simulink model "SingleTrackCANoe"  (R2021b)
settings: Solver=ode1  StartTime=0  StopTime=2  FixedStep=1.0000000000000000e-003  RelTol=1e-3
InitFcn:
  | sampleTime = str2double(get_param(bdroot, 'FixedStep'));
undefined symbols (not defined in the file or in its folder): AccPedalPos, BrakePedalPos, BrakeSwitch, DiscIntNeverNeededParam, DYNA4, EngSpd, IgnitionSwitch, InitialGear, InitialSpeed, IntendedEngTrq, LeftIndicator, MainBrakePress, MaxGear, MDL, MinGear, RefAcc, RefLane, RefLatPos, RefPath, RefPathCurv, RefSpd, RefSpdPreview, RefSpdRetrospect, RightIndicator, SteeringWheelAng, SteeringWheelTrq, UserDefinedRefValue, vm_const
libraries: UtilitiesLibrary x62, simulink x18, WheelSystemModules x14, LongitudinalControllerModules x13, LateralControllerModules x7, AnimationBusselectorModules x5, EnvironmentModules x5, BasicEngineControlModules x5, MiscellaneousControlModules x5, Animation3Modules x4, AuxiliariesModules x4, ReducedTireModules x4
(part 10 of 34)

== system SingleTrackCANoe/SimulationModel/VehicleControl/VehicleControlOutput ==
  InitialConditions___UNIQUE_1 : Inport  Description=|
      | <name>InitialConditions</name>
      | <comment></comment>
  LongitudinalControl___UNIQUE_1 : Inport  Description=|  Port=2
      | <name>LongitudinalControl</name>
      | <comment></comment>
  LateralControl___UNIQUE_1 : Inport  Description=|  Port=3
      | <name>LateralControl</name>
      | <comment></comment>
  BrakeHydraulicsControl___UNIQUE_1 : Inport  Description=|  Port=4
      | <name>BrakeHydraulicsControl</name>
      | <comment></comment>
  EngineControl___UNIQUE_1 : Inport  Description=|  Port=5
      | <name>EngineControl</name>
      | <comment></comment>
  SuspensionTestRigControl___UNIQUE_1 : Inport  Description=|  Port=6
      | <name>SuspensionTestRigControl</name>
      | <comment></comment>
  TemperatureControl___UNIQUE_1 : Inport  Description=|  Port=7
      | <name>TemperatureControl</name>
      | <comment></comment>
  UserDefinedControl___UNIQUE_1 : Inport  Description=|  Port=8
      | <name>UserDefinedControl</name>
      | <comment></comment>
  __TDO__VehicleControl : BusCreator  Inputs=8
  VehicleControl___UNIQUE_1 : Outport  Description=|  VectorParamsAs1DForOutWhenUnconnected=off
      | <name>InitialConditions</name>
      | <comment></comment>
  wires:
  InitialConditions___UNIQUE_1/1 -> __TDO__VehicleControl/1  "InitialConditions"
  LongitudinalControl___UNIQUE_1/1 -> __TDO__VehicleControl/2  "LongitudinalControl"
  LateralControl___UNIQUE_1/1 -> __TDO__VehicleControl/3  "LateralControl"
  BrakeHydraulicsControl___UNIQUE_1/1 -> __TDO__VehicleControl/4  "BrakeHydraulicsControl"
  EngineControl___UNIQUE_1/1 -> __TDO__VehicleControl/5  "EngineControl"
  SuspensionTestRigControl___UNIQUE_1/1 -> __TDO__VehicleControl/6  "SuspensionTestRigControl"
  TemperatureControl___UNIQUE_1/1 -> __TDO__VehicleControl/7  "TemperatureControl"
  UserDefinedControl___UNIQUE_1/1 -> __TDO__VehicleControl/8  "UserDefinedControl"
  __TDO__VehicleControl/1 -> VehicleControl___UNIQUE_1/1  "VehicleControl"

== system SingleTrackCANoe/SimulationModel/ControlUnits/ADAS/ADASOutput ==
  __SRC__ADAS.LongitudinalControlIntervention[0;1] : Constant  Value=0.0  OutDataTypeStr=Inherit: Inherit via back propagation
  __SRC__ADAS.PrioritizedADASControl.LimitsActive[0;1] : Constant  Value=0.0  OutDataTypeStr=Inherit: Inherit via back propagation
  __SRC__ADAS.PrioritizedADASControl.LowerLimitBrakePress[Pa] : Constant  Value=0.0  OutDataTypeStr=Inherit: Inherit via back propagation
  __SRC__ADAS.PrioritizedADASControl.LowerLimitTrq[Nm] : Constant  Value=-vm_const('PAR_NOT_GIVEN')  OutDataTypeStr=Inherit: Inherit via back propagation
  __SRC__ADAS.PrioritizedADASControl.UpperLimitTrq[Nm] : Constant  Value=vm_const('PAR_NOT_GIVEN')  OutDataTypeStr=Inherit: Inherit via back propagation
  __TDO__ADAS : BusCreator  Inputs=2
  __TDO__ADAS.PrioritizedADASControl : BusCreator  Inputs=4
  ADAS___UNIQUE_1 : Outport  Description=|  PortDimensions=[5]  VectorParamsAs1DForOutWhenUnconnected=off
      | <name>PrioritizedADASControl.LimitsActive[0;1]</name>
      | <comment></comment>
  wires:
  __SRC__ADAS.PrioritizedADASControl.LimitsActive[0;1]/1 -> __TDO__ADAS.PrioritizedADASControl/1  "LimitsActive[0;1]"
  __TDO__ADAS.PrioritizedADASControl/1 -> __TDO__ADAS/1  "PrioritizedADASControl"
  __SRC__ADAS.PrioritizedADASControl.UpperLimitTrq[Nm]/1 -> __TDO__ADAS.PrioritizedADASControl/2  "UpperLimitTrq[Nm]"
  __SRC__ADAS.PrioritizedADASControl.LowerLimitTrq[Nm]/1 -> __TDO__ADAS.PrioritizedADASControl/3  "LowerLimitTrq[Nm]"
  __SRC__ADAS.PrioritizedADASControl.LowerLimitBrakePress[Pa]/1 -> __TDO__ADAS.PrioritizedADASControl/4  "LowerLimitBrakePress[Pa]"
  __SRC__ADAS.LongitudinalControlIntervention[0;1]/1 -> __TDO__ADAS/2  "LongitudinalControlIntervention[0;1]"
  __TDO__ADAS/1 -> ADAS___UNIQUE_1/1  "ADAS"

== system SingleTrackCANoe/SimulationModel/ControlUnits/ADAS/DynaComponentInfo ==

== system SingleTrackCANoe/SimulationModel/ControlUnits/LCU/DynaComponentInfo ==

== system SingleTrackCANoe/SimulationModel/ControlUnits/LCU/LCUOutput ==
  VehicleLights___UNIQUE_1 : Inport  Description=|
      | <name>VehicleLights</name>
      | <comment></comment>
  __TDO__LCU : BusCreator  Inputs=1
  LCU___UNIQUE_1 : Outport  Description=|  VectorParamsAs1DForOutWhenUnconnected=off
      | <name>VehicleLights</name>
      | <comment></comment>
  wires:
  VehicleLights___UNIQUE_1/1 -> __TDO__LCU/1  "VehicleLights"
  __TDO__LCU/1 -> LCU___UNIQUE_1/1  "LCU"

== system SingleTrackCANoe/SimulationModel/ControlUnits/StateSensors/DynaComponentInfo ==

== system SingleTrackCANoe/SimulationModel/ControlUnits/StateSensors/StateSensorsOutput ==
  IMU___UNIQUE_1 : Inport  Description=|
      | <name>IMU</name>
      | <comment></comment>
  __TDO__StateSensors : BusCreator  Inputs=1
  StateSensors___UNIQUE_1 : Outport  Description=|  VectorParamsAs1DForOutWhenUnconnected=off
      | <name>IMU</name>
      | <comment></comment>
  wires:
  IMU___UNIQUE_1/1 -> __TDO__StateSensors/1  "IMU"
  __TDO__StateSensors/1 -> StateSensors___UNIQUE_1/1  "StateSensors"

== system SingleTrackCANoe/SimulationModel/ControlUnits/VCU/DynaComponentInfo ==

== system SingleTrackCANoe/SimulationModel/ControlUnits/VCU/InputFromADAS ==
  fromADAS : Inport  Description=|
      | <name>DriverBrakePedalMode[0;1;2]</name>
      | <comment></comment>
  TDBusSelector : BusSelector  OutputSignals=PrioritizedADASControl
  __TDO__PrioritizedADASControl : BusCreator  Inputs=1
  PrioritizedADASControl___UNIQUE_1 : Outport  Description=|
      | <name>PrioritizedADASControl</name>
      | <comment></comment>
  wires:
  fromADAS/1 -> TDBusSelector/1  "ControlSignals"
  TDBusSelector/1 -> __TDO__PrioritizedADASControl/1  "<PrioritizedADASControl>"
  __TDO__PrioritizedADASControl/1 -> PrioritizedADASControl___UNIQUE_1/1  "PrioritizedADASControl"

== system SingleTrackCANoe/SimulationModel/ControlUnits/VCU/InputFromCTRL ==
  fromCTRL : Inport
  TDBusSelector : BusSelector  OutputSignals=CTRL.LongitudinalControl.AccPedalPos[0_1],CTRL.LongitudinalControl.BrakePedalPos[0_1],CTRL.LongitudinalControl.DriverInfo.MeanEngMaxTrq[Nm],CTRL.LongitudinalControl.DriverInfo.MeanEngDragTrq[Nm],CTRL.LongitudinalControl.DriverInfo.ThirtyPercentAccPedalEngTrq[Nm]
  __TDD__AccPedalPos[0_1] : Demux  Outputs=[1]
  __TDD__BrakePedalPos[0_1] : Demux  Outputs=1
  __TDD__MeanEngDragTrq[Nm] : Demux  Outputs=[1]
  __TDD__MeanEngMaxTrq[Nm] : Demux  Outputs=[1]
  __TDD__ThirtyPercentAccPedalEngTrq[Nm] : Demux  Outputs=[1]
  AccPedalPos[0_1] : Outport  Description=|  PortDimensions=[1]  VectorParamsAs1DForOutWhenUnconnected=off
      | <name>CTRL.LongitudinalControl.AccPedalPos[0_1]</name>
      | <comment>Accelerator pedal position</comment>
  BrakePedalPos[0_1]___UNIQUE_1 : Outport  Description=|  Port=2  VectorParamsAs1DForOutWhenUnconnected=off
      | <name>CTRL.LongitudinalControl.BrakePedalPos[0_1]</name>
      | <comment></comment>
  MeanEngMaxTrq[Nm]___UNIQUE_1 : Outport  Description=|  Port=3  PortDimensions=[1]  VectorParamsAs1DForOutWhenUnconnected=off
      | <name>CTRL.LongitudinalControl.DriverInfo.MeanEngMaxTrq[Nm]</name>
      | <comment></comment>
  MeanEngDragTrq[Nm]___UNIQUE_1 : Outport  Description=|  Port=4  PortDimensions=[1]  VectorParamsAs1DForOutWhenUnconnected=off
      | <name>CTRL.LongitudinalControl.DriverInfo.MeanEngDragTrq[Nm]</name>
      | <comment></comment>
  ThirtyPercentAccPedalEngTrq[Nm]___UNIQUE_1 : Outport  Description=|  Port=5  PortDimensions=[1]
      | <name>CTRL.LongitudinalControl.DriverInfo.ThirtyPercentAccPedalEngTrq[Nm]</name>
      | <comment></comment>
  wires:
  __TDD__ThirtyPercentAccPedalEngTrq[Nm]/1 -> ThirtyPercentAccPedalEngTrq[Nm]___UNIQUE_1/1  "ThirtyPercentAccPedalEngTrq[Nm]"
  __TDD__MeanEngDragTrq[Nm]/1 -> MeanEngDragTrq[Nm]___UNIQUE_1/1  "MeanEngDragTrq[Nm]"
  __TDD__MeanEngMaxTrq[Nm]/1 -> MeanEngMaxTrq[Nm]___UNIQUE_1/1  "MeanEngMaxTrq[Nm]"
  __TDD__BrakePedalPos[0_1]/1 -> BrakePedalPos[0_1]___UNIQUE_1/1  "BrakePedalPos[0_1]"
  __TDD__AccPedalPos[0_1]/1 -> AccPedalPos[0_1]/1  "AccPedalPos[0_1]"
  TDBusSelector/5 -> __TDD__ThirtyPercentAccPedalEngTrq[Nm]/1  "<ThirtyPercentAccPedalEngTrq[Nm]>"
  TDBusSelector/4 -> __TDD__MeanEngDragTrq[Nm]/1  "<MeanEngDragTrq[Nm]>"
  TDBusSelector/3 -> __TDD__MeanEngMaxTrq[Nm]/1  "<MeanEngMaxTrq[Nm]>"
  TDBusSelector/2 -> __TDD__BrakePedalPos[0_1]/1  "<BrakePedalPos[0_1]>"
  TDBusSelector/1 -> __TDD__AccPedalPos[0_1]/1  "<AccPedalPos[0_1]>"
  fromCTRL/1 -> TDBusSelector/1

== system SingleTrackCANoe/SimulationModel/ControlUnits/VCU/InputFromVehicle ==
  fromVehicle : Inport
  TDBusSelector : BusSelector  OutputSignals=BrakeSystem.BrakeSystemPhysics.MaxMainBrakePress[Pa]
  __TDD__MaxMainBrakePress[Pa] : Demux  Outputs=[1]
  MaxMainBrakePress[Pa]___UNIQUE_1 : Outport  Description=|  PortDimensions=[1]  VectorParamsAs1DForOutWhenUnconnected=off
      | <name>BrakeSystem.BrakeSystemPhysics.MaxMainBrakePress[Pa]</name>
      | <comment>Maximum main brake pressure</comment>
  wires:
  fromVehicle/1 -> TDBusSelector/1
  TDBusSelector/1 -> __TDD__MaxMainBrakePress[Pa]/1  "<MaxMainBrakePress[Pa]>"
  __TDD__MaxMainBrakePress[Pa]/1 -> MaxMainBrakePress[Pa]___UNIQUE_1/1  "MaxMainBrakePress[Pa]"

== system SingleTrackCANoe/SimulationModel/ControlUnits/VCU/VCUOutput ==
  TransmissionLoad[0_1]___UNIQUE_1 : Inport  Description=|  PortDimensions=[1]
      | <name>TransmissionLoad[0_1]</name>
      | <comment></comment>
  IntendedEngTrq[Nm]___UNIQUE_1 : Inport  Description=|  Port=2  PortDimensions=[1]
      | <name>IntendedEngTrq[Nm]</name>
      | <comment>Intended torque of engine</comment>
  IntendedEngTrqActive[0;1]___UNIQUE_1 : Inport  Description=|  Port=3  PortDimensions=[1]
      | <name>IntendedEngTrqActive[0;1]</name>
      | <comment></comment>
  IntendedMainBrakePress[Pa]___UNIQUE_1 : Inport  Description=|  Port=4  PortDimensions=[1]
      | <name>IntendedMainBrakePress[Pa]</name>
      | <comment></comment>
  IntendedMainBrakePressActive[0;1]___UNIQUE_1 : Inport  Description=|  Port=5  PortDimensions=[1]
      | <name>IntendedMainBrakePressActive[0;1]</name>
      | <comment></comment>
  __SAT__VCU.EngRunPermission[0;1] : Saturate  UpperLimit=1  LowerLimit=0
  __SRC__VCU.DriverInfo.ConventionalVehicleSwitch[0;1] : Constant  Value=1.0  OutDataTypeStr=Inherit: Inherit via back propagation
  __SRC__VCU.DrivingState[-] : Constant  Value=0.0  OutDataTypeStr=Inherit: Inherit via back propagation
  __SRC__VCU.EngRunPermission[0;1] : Constant  Value=1.0  OutDataTypeStr=Inherit: Inherit via back propagation
  __TDD__VCU.IntendedEngTrqActive[0;1] : Demux  Outputs=[1]
  __TDD__VCU.IntendedEngTrq[Nm] : Demux  Outputs=[1]
  __TDD__VCU.IntendedMainBrakePressActive[0;1] : Demux  Outputs=[1]
  __TDD__VCU.IntendedMainBrakePress[Pa] : Demux  Outputs=[1]
  __TDD__VCU.TransmissionLoad[0_1] : Demux  Outputs=[1]
  __TDO__VCU : BusCreator  Inputs=8
  __TDO__VCU.DriverInfo : BusCreator  Inputs=1
  VCU___UNIQUE_1 : Outport  Description=|  PortDimensions=[8]  VectorParamsAs1DForOutWhenUnconnected=off
      | <name>TransmissionLoad[0_1]</name>
      | <comment></comment>
  wires:
  __SRC__VCU.EngRunPermission[0;1]/1 -> __SAT__VCU.EngRunPermission[0;1]/1
  TransmissionLoad[0_1]___UNIQUE_1/1 -> __TDD__VCU.TransmissionLoad[0_1]/1
  __TDD__VCU.TransmissionLoad[0_1]/1 -> __TDO__VCU/1  "TransmissionLoad[0_1]"
  IntendedEngTrq[Nm]___UNIQUE_1/1 -> __TDD__VCU.IntendedEngTrq[Nm]/1
  __TDD__VCU.IntendedEngTrq[Nm]/1 -> __TDO__VCU/2  "IntendedEngTrq[Nm]"
  IntendedEngTrqActive[0;1]___UNIQUE_1/1 -> __TDD__VCU.IntendedEngTrqActive[0;1]/1
  __TDD__VCU.IntendedEngTrqActive[0;1]/1 -> __TDO__VCU/3  "IntendedEngTrqActive[0;1]"
  IntendedMainBrakePress[Pa]___UNIQUE_1/1 -> __TDD__VCU.IntendedMainBrakePress[Pa]/1
  __TDD__VCU.IntendedMainBrakePress[Pa]/1 -> __TDO__VCU/4  "IntendedMainBrakePress[Pa]"
  IntendedMainBrakePressActive[0;1]___UNIQUE_1/1 -> __TDD__VCU.IntendedMainBrakePressActive[0;1]/1
  __TDD__VCU.IntendedMainBrakePressActive[0;1]/1 -> __TDO__VCU/5  "IntendedMainBrakePressActive[0;1]"
  __SRC__VCU.DrivingState[-]/1 -> __TDO__VCU/6  "DrivingState[-]"
  __SRC__VCU.DriverInfo.ConventionalVehicleSwitch[0;1]/1 -> __TDO__VCU.DriverInfo/1  "ConventionalVehicleSwitch[0;1]"
  __TDO__VCU.DriverInfo/1 -> __TDO__VCU/7  "DriverInfo"
  __SAT__VCU.EngRunPermission[0;1]/1 -> __TDO__VCU/8  "EngRunPermission[0;1]"
  __TDO__VCU/1 -> VCU___UNIQUE_1/1  "VCU"

== system SingleTrackCANoe/SimulationModel/Environment/Road/DynaSystemInfo ==

== system SingleTrackCANoe/SimulationModel/Traffic/TrafficOutputs/DistanceToVehicleOutput ==
  LeftAdjacentLaneFrontalDist[m]___UNIQUE_1 : Inport  Description=|  PortDimensions=[1]
      | <name>LeftAdjacentLaneFrontalDist[m]</name>
      | <comment>Distance of VuT to next frontal traffic object on left adjacent lane</comment>
  LeftAdjacentLaneRearDist[m]___UNIQUE_1 : Inport  Description=|  Port=2  PortDimensions=[1]
      | <name>LeftAdjacentLaneRearDist[m]</name>
      | <comment>Distance of VuT to next rear traffic object on left adjacent lane</comment>
  MyLaneFrontalDist[m]___UNIQUE_1 : Inport  Description=|  Port=3  PortDimensions=[1]
      | <name>MyLaneFrontalDist[m]</name>
      | <comment>Distance of VuT to next frontal traffic object on the same lane</comment>
  MyLaneRearDist[m]___UNIQUE_1 : Inport  Description=|  Port=4  PortDimensions=[1]
      | <name>MyLaneRearDist[m]</name>
      | <comment>Distance of VuT to next rear traffic object on the same lane</comment>
  RightAdjacentLaneFrontalDist[m]___UNIQUE_1 : Inport  Description=|  Port=5  PortDimensions=[1]
      | <name>RightAdjacentLaneFrontalDist[m]</name>
      | <comment>Distance of VuT to next frontal traffic object on right adjacent lane</comment>
  RightAdjacentLaneRearDist[m]___UNIQUE_1 : Inport  Description=|  Port=6  PortDimensions=[1]
      | <name>RightAdjacentLaneRearDist[m]</name>
      | <comment>Distance of VuT to next rear traffic object on right adjacent lane</comment>
  LeftAdjacentLaneFrontalSpd[m/s]___UNIQUE_1 : Inport  Description=|  Port=7  PortDimensions=[1]
      | <name>LeftAdjacentLaneFrontalSpd[m/s]</name>
      | <comment>Longitudinal speed of next frontal traffic object on left adjacent lane</comment>
  LeftAdjacentLaneRearSpd[m/s]___UNIQUE_1 : Inport  Description=|  Port=8  PortDimensions=[1]
      | <name>LeftAdjacentLaneRearSpd[m/s]</name>
      | <comment>Longitudinal speed of next rear traffic object on left adjacent lane</comment>
  MyLaneFrontalSpd[m/s]___UNIQUE_1 : Inport  Description=|  Port=9  PortDimensions=[1]
      | <name>MyLaneFrontalSpd[m/s]</name>
      | <comment>Longitudinal speed of next frontal traffic object on the same lane</comment>
  MyLaneRearSpd[m/s]___UNIQUE_1 : Inport  Description=|  Port=10  PortDimensions=[1]
      | <name>MyLaneRearSpd[m/s]</name>
      | <comment>Longitudinal speed of next rear traffic object on the same lane</comment>
  RightAdjacentLaneFrontalSpd[m/s]___UNIQUE_1 : Inport  Description=|  Port=11  PortDimensions=[1]
      | <name>RightAdjacentLaneFrontalSpd[m/s]</name>
      | <comment>Longitudinal speed of next frontal traffic object on right adjacent lane</comment>
  RightAdjacentLaneRearSpd[m/s]___UNIQUE_1 : Inport  Description=|  Port=12  PortDimensions=[1]
      | <name>RightAdjacentLaneRearSpd[m/s]</name>
      | <comment>Longitudinal speed of next rear traffic object on right adjacent lane</comment>
  __TDD__Traffic.AdjacentObjectsSpeeds.LeftAdjacentLaneFrontalSpd[m/s] : Demux  Outputs=[1]
  __TDD__Traffic.AdjacentObjectsSpeeds.LeftAdjacentLaneRearSpd[m/s] : Demux  Outputs=[1]
  __TDD__Traffic.AdjacentObjectsSpeeds.MyLaneFrontalSpd[m/s] : Demux  Outputs=[1]
  __TDD__Traffic.AdjacentObjectsSpeeds.MyLaneRearSpd[m/s] : Demux  Outputs=[1]
  __TDD__Traffic.AdjacentObjectsSpeeds.RightAdjacentLaneFrontalSpd[m/s] : Demux  Outputs=[1]
  __TDD__Traffic.AdjacentObjectsSpeeds.RightAdjacentLaneRearSpd[m/s] : Demux  Outputs=[1]
  __TDD__Traffic.DistancesToVehicle.LeftAdjacentLaneFrontalDist[m] : Demux  Outputs=[1]
  __TDD__Traffic.DistancesToVehicle.LeftAdjacentLaneRearDist[m] : Demux  Outputs=[1]
  __TDD__Traffic.DistancesToVehicle.MyLaneFrontalDist[m] : Demux  Outputs=[1]
  __TDD__Traffic.DistancesToVehicle.MyLaneRearDist[m] : Demux  Outputs=[1]
  __TDD__Traffic.DistancesToVehicle.RightAdjacentLaneFrontalDist[m] : Demux  Outputs=[1]
  __TDD__Traffic.DistancesToVehicle.RightAdjacentLaneRearDist[m] : Demux  Outputs=[1]
  __TDO__Traffic : BusCreator  Inputs=2
  __TDO__Traffic.AdjacentObjectsSpeeds : BusCreator  Inputs=6
  __TDO__Traffic.DistancesToVehicle : BusCreator  Inputs=6
  Traffic___UNIQUE_1 : Outport  Description=|  PortDimensions=[12]  VectorParamsAs1DForOutWhenUnconnected=off
      | <name>LeftAdjacentLaneFrontalDist[m]</name>
      | <comment>Distance of VuT to next frontal traffic object on left adjacent lane</comment>
  wires:
  LeftAdjacentLaneFrontalDist[m]___UNIQUE_1/1 -> __TDD__Traffic.DistancesToVehicle.LeftAdjacentLaneFrontalDist[m]/1
  __TDD__Traffic.DistancesToVehicle.LeftAdjacentLaneFrontalDist[m]/1 -> __TDO__Traffic.DistancesToVehicle/1  "LeftAdjacentLaneFrontalDist[m]"
  __TDO__Traffic.DistancesToVehicle/1 -> __TDO__Traffic/1  "DistancesToVehicle"
  LeftAdjacentLaneRearDist[m]___UNIQUE_1/1 -> __TDD__Traffic.DistancesToVehicle.LeftAdjacentLaneRearDist[m]/1
  __TDD__Traffic.DistancesToVehicle.LeftAdjacentLaneRearDist[m]/1 -> __TDO__Traffic.DistancesToVehicle/2  "LeftAdjacentLaneRearDist[m]"
  MyLaneFrontalDist[m]___UNIQUE_1/1 -> __TDD__Traffic.DistancesToVehicle.MyLaneFrontalDist[m]/1
  __TDD__Traffic.DistancesToVehicle.MyLaneFrontalDist[m]/1 -> __TDO__Traffic.DistancesToVehicle/3  "MyLaneFrontalDist[m]"
  MyLaneRearDist[m]___UNIQUE_1/1 -> __TDD__Traffic.DistancesToVehicle.MyLaneRearDist[m]/1
  __TDD__Traffic.DistancesToVehicle.MyLaneRearDist[m]/1 -> __TDO__Traffic.DistancesToVehicle/4  "MyLaneRearDist[m]"
  RightAdjacentLaneFrontalDist[m]___UNIQUE_1/1 -> __TDD__Traffic.DistancesToVehicle.RightAdjacentLaneFrontalDist[m]/1
  __TDD__Traffic.DistancesToVehicle.RightAdjacentLaneFrontalDist[m]/1 -> __TDO__Traffic.DistancesToVehicle/5  "RightAdjacentLaneFrontalDist[m]"
  RightAdjacentLaneRearDist[m]___UNIQUE_1/1 -> __TDD__Traffic.DistancesToVehicle.RightAdjacentLaneRearDist[m]/1
  __TDD__Traffic.DistancesToVehicle.RightAdjacentLaneRearDist[m]/1 -> __TDO__Traffic.DistancesToVehicle/6  "RightAdjacentLaneRearDist[m]"
  LeftAdjacentLaneFrontalSpd[m/s]___UNIQUE_1/1 -> __TDD__Traffic.AdjacentObjectsSpeeds.LeftAdjacentLaneFrontalSpd[m/s]/1
  __TDD__Traffic.AdjacentObjectsSpeeds.LeftAdjacentLaneFrontalSpd[m/s]/1 -> __TDO__Traffic.AdjacentObjectsSpeeds/1  "LeftAdjacentLaneFrontalSpd[m/s]"
  __TDO__Traffic.AdjacentObjectsSpeeds/1 -> __TDO__Traffic/2  "AdjacentObjectsSpeeds"
  LeftAdjacentLaneRearSpd[m/s]___UNIQUE_1/1 -> __TDD__Traffic.AdjacentObjectsSpeeds.LeftAdjacentLaneRearSpd[m/s]/1
  __TDD__Traffic.AdjacentObjectsSpeeds.LeftAdjacentLaneRearSpd[m/s]/1 -> __TDO__Traffic.AdjacentObjectsSpeeds/2  "LeftAdjacentLaneRearSpd[m/s]"
  MyLaneFrontalSpd[m/s]___UNIQUE_1/1 -> __TDD__Traffic.AdjacentObjectsSpeeds.MyLaneFrontalSpd[m/s]/1
  __TDD__Traffic.AdjacentObjectsSpeeds.MyLaneFrontalSpd[m/s]/1 -> __TDO__Traffic.AdjacentObjectsSpeeds/3  "MyLaneFrontalSpd[m/s]"
  MyLaneRearSpd[m/s]___UNIQUE_1/1 -> __TDD__Traffic.AdjacentObjectsSpeeds.MyLaneRearSpd[m/s]/1
  __TDD__Traffic.AdjacentObjectsSpeeds.MyLaneRearSpd[m/s]/1 -> __TDO__Traffic.AdjacentObjectsSpeeds/4  "MyLaneRearSpd[m/s]"
  RightAdjacentLaneFrontalSpd[m/s]___UNIQUE_1/1 -> __TDD__Traffic.AdjacentObjectsSpeeds.RightAdjacentLaneFrontalSpd[m/s]/1
  __TDD__Traffic.AdjacentObjectsSpeeds.RightAdjacentLaneFrontalSpd[m/s]/1 -> __TDO__Traffic.AdjacentObjectsSpeeds/5  "RightAdjacentLaneFrontalSpd[m/s]"
  RightAdjacentLaneRearSpd[m/s]___UNIQUE_1/1 -> __TDD__Traffic.AdjacentObjectsSpeeds.RightAdjacentLaneRearSpd[m/s]/1
  __TDD__Traffic.AdjacentObjectsSpeeds.RightAdjacentLaneRearSpd[m/s]/1 -> __TDO__Traffic.AdjacentObjectsSpeeds/6  "RightAdjacentLaneRearSpd[m/s]"
  __TDO__Traffic/1 -> Traffic___UNIQUE_1/1  "Traffic"

== system SingleTrackCANoe/SimulationModel/Vehicle/Auxiliaries/AuxiliariesOutput ==
  GeneratorCurr[A]___UNIQUE_1 : Inport  Description=|  PortDimensions=[1]
      | <name>GeneratorCurr[A]</name>
      | <comment></comment>
  GeneratorTrq[Nm]___UNIQUE_1 : Inport  Description=|  Port=2  PortDimensions=[1]
      | <name>GeneratorTrq[Nm]</name>
      | <comment></comment>
  GeneratorInrt[kgm^2]___UNIQUE_1 : Inport  Description=|  Port=3  PortDimensions=[1]
      | <name>GeneratorInrt[kgm^2]</name>
      | <comment></comment>
  StarterCurr[A]___UNIQUE_1 : Inport  Description=|  Port=4  PortDimensions=[1]
      | <name>StarterCurr[A]</name>
      | <comment></comment>
  StarterTrq[Nm]___UNIQUE_1 : Inport  Description=|  Port=5  PortDimensions=[1]
      | <name>StarterTrq[Nm]</name>
      | <comment></comment>
  StarterInrt[kgm**2]___UNIQUE_1 : Inport  Description=|  Port=6  PortDimensions=[1]
      | <name>StarterInrt[kgm**2]</name>
      | <comment></comment>
  __TDD__Auxiliaries.GeneratorCurr[A] : Demux  Outputs=[1]
  __TDD__Auxiliaries.GeneratorInrt[kgm^2] : Demux  Outputs=[1]
  __TDD__Auxiliaries.GeneratorTrq[Nm] : Demux  Outputs=[1]
  __TDD__Auxiliaries.StarterCurr[A] : Demux  Outputs=[1]
  __TDD__Auxiliaries.StarterInrt[kgm**2] : Demux  Outputs=[1]
  __TDD__Auxiliaries.StarterTrq[Nm] : Demux  Outputs=[1]
  __TDO__Auxiliaries : BusCreator  Inputs=6
  Auxiliaries___UNIQUE_1 : Outport  Description=|  PortDimensions=[6]  VectorParamsAs1DForOutWhenUnconnected=off
      | <name>GeneratorCurr[A]</name>
      | <comment></comment>
  wires:
  __TDO__Auxiliaries/1 -> Auxiliaries___UNIQUE_1/1  "Auxiliaries"
  __TDD__Auxiliaries.StarterInrt[kgm**2]/1 -> __TDO__Auxiliaries/6  "StarterInrt[kgm**2]"
  StarterInrt[kgm**2]___UNIQUE_1/1 -> __TDD__Auxiliaries.StarterInrt[kgm**2]/1
  __TDD__Auxiliaries.StarterTrq[Nm]/1 -> __TDO__Auxiliaries/5  "StarterTrq[Nm]"
  StarterTrq[Nm]___UNIQUE_1/1 -> __TDD__Auxiliaries.StarterTrq[Nm]/1
  __TDD__Auxiliaries.StarterCurr[A]/1 -> __TDO__Auxiliaries/4  "StarterCurr[A]"
  StarterCurr[A]___UNIQUE_1/1 -> __TDD__Auxiliaries.StarterCurr[A]/1
  __TDD__Auxiliaries.GeneratorInrt[kgm^2]/1 -> __TDO__Auxiliaries/3  "GeneratorInrt[kgm^2]"
  GeneratorInrt[kgm^2]___UNIQUE_1/1 -> __TDD__Auxiliaries.GeneratorInrt[kgm^2]/1
  __TDD__Auxiliaries.GeneratorTrq[Nm]/1 -> __TDO__Auxiliaries/2  "GeneratorTrq[Nm]"
  GeneratorTrq[Nm]___UNIQUE_1/1 -> __TDD__Auxiliaries.GeneratorTrq[Nm]/1
  __TDD__Auxiliaries.GeneratorCurr[A]/1 -> __TDO__Auxiliaries/1  "GeneratorCurr[A]"
  GeneratorCurr[A]___UNIQUE_1/1 -> __TDD__Auxiliaries.GeneratorCurr[A]/1

== system SingleTrackCANoe/SimulationModel/Vehicle/Auxiliaries/DynaComponentInfo ==

== system SingleTrackCANoe/SimulationModel/Vehicle/Auxiliaries/Generator ==
  EngSpd [rad/s] : Inport
  GeneratorVoltage [V] : Inport  Port=2
  RefVoltage [V] : Inport  Port=3
  LRTime [s] : Inport  Port=4
  Temp [K] : Inport  Port=5
  BattVoltage [V] : Inport  Port=6
  Alternator : AuxiliariesModules/Alternator  DATA_NODE=MDL.Vehicle.Auxiliaries.Alternator  trq_table=MDL.Vehicle.Auxiliaries.Alternator.TrqMap  max_current=MDL.Vehicle.Auxiliaries.Alternator.MaxCurrMap  max_current_rate=MDL.Vehicle.Auxiliaries.Alternator.MaxCurrRate  ref_volt=MDL.Vehicle.Auxiliaries.Alternator.RefVoltage  resist=MDL.Vehicle.Auxiliaries.Alternator.Resist  ratio=MDL.Vehicle.Auxiliaries.Alternator.SpdRatio  Inrt=MDL.Vehicle.Auxiliaries.Alternator.Inrt
  InitCurr [A] : Constant  Value=0
  VoltageRegulator : AuxiliariesModules/VoltageRegulator  DATA_NODE=MDL.Vehicle.Auxiliaries.VoltageRegulator  min_lr=MDL.Vehicle.Auxiliaries.VoltageRegulator.MinLoadResponseTime  LR_thres=MDL.Vehicle.Auxiliaries.VoltageRegulator.LoadResponseSpdLimit
  Curr [A] : Outport  VectorParamsAs1DForOutWhenUnconnected=off
  Trq [Nm] : Outport  Port=2  VectorParamsAs1DForOutWhenUnconnected=off
  Inrt [kgm**2] : Outport  Port=3  VectorParamsAs1DForOutWhenUnconnected=off
  wires:
  VoltageRegulator/1 -> Alternator/1
  EngSpd [rad/s]/1 -> VoltageRegulator/1, Alternator/2
  GeneratorVoltage [V]/1 -> Alternator/3
  InitCurr [A]/1 -> VoltageRegulator/5
  Alternator/4 -> VoltageRegulator/6
  RefVoltage [V]/1 -> VoltageRegulator/3
  LRTime [s]/1 -> VoltageRegulator/4
  Alternator/1 -> Curr [A]/1
  Alternator/2 -> Trq [Nm]/1
  Alternator/3 -> Inrt [kgm**2]/1
  Temp [K]/1 -> Alternator/4
  BattVoltage [V]/1 -> VoltageRegulator/2

== system SingleTrackCANoe/SimulationModel/Vehicle/Auxiliaries/InputFromCTRL ==
  fromCTRL : Inport
  TDBusSelector : BusSelector  OutputSignals=CTRL.LongitudinalControl.StarterSwitch[0;1],CTRL.EnvironmentalConditions.AmbTemp[K]
  __TDD__AmbTemp[K] : Demux  Outputs=[1]
  __TDD__StarterSwitch[0;1] : Demux  Outputs=[1]
  StarterSwitch[0;1]___UNIQUE_1 : Outport  Description=|  PortDimensions=[1]  VectorParamsAs1DForOutWhenUnconnected=off
      | <name>CTRL.LongitudinalControl.StarterSwitch[0;1]</name>
      | <comment>Engine starter switch</comment>
  AmbTemp[K]___UNIQUE_1 : Outport  Description=|  Port=2  PortDimensions=[1]  VectorParamsAs1DForOutWhenUnconnected=off
      | <name>CTRL.EnvironmentalConditions.AmbTemp[K]</name>
      | <comment></comment>
  wires:
  __TDD__AmbTemp[K]/1 -> AmbTemp[K]___UNIQUE_1/1  "AmbTemp[K]"
  __TDD__StarterSwitch[0;1]/1 -> StarterSwitch[0;1]___UNIQUE_1/1  "StarterSwitch[0;1]"
  TDBusSelector/2 -> __TDD__AmbTemp[K]/1  "<AmbTemp[K]>"
  TDBusSelector/1 -> __TDD__StarterSwitch[0;1]/1  "<StarterSwitch[0;1]>"
  fromCTRL/1 -> TDBusSelector/1

== system SingleTrackCANoe/SimulationModel/Vehicle/Auxiliaries/InputFromDrivetrain ==
  fromDrivetrain : Inport
  TDBusSelector : BusSelector  OutputSignals=DrivetrainPhysics.EngSpd[rad/s]
  __TDD__EngSpd[rad/s] : Demux  Outputs=1
  EngSpd[rad/s] : Outport  Description=|  VectorParamsAs1DForOutWhenUnconnected=off
      | <name>DrivetrainPhysics.EngSpd[rad/s]</name>
      | <comment></comment>
  wires:
  __TDD__EngSpd[rad/s]/1 -> EngSpd[rad/s]/1  "EngSpd[rad/s]"
  TDBusSelector/1 -> __TDD__EngSpd[rad/s]/1  "<EngSpd[rad/s]>"
  fromDrivetrain/1 -> TDBusSelector/1

== system SingleTrackCANoe/SimulationModel/Vehicle/Auxiliaries/InputFromElectricalSystem ==
  fromPowernet : Inport
  TDBusSelector : BusSelector  OutputSignals=GeneratorVoltage[V],LowVoltageBattery.LowVoltageBatteryVoltage[V],StarterVoltage[V]
  __TDD__GeneratorVoltage[V] : Demux  Outputs=[1]
  __TDD__LowVoltageBatteryVoltage[V] : Demux  Outputs=[1]
  __TDD__StarterVoltage[V] : Demux  Outputs=[1]
  GeneratorVoltage[V]___UNIQUE_1 : Outport  Description=|  PortDimensions=[1]  VectorParamsAs1DForOutWhenUnconnected=off
      | <name>GeneratorVoltage[V]</name>
      | <comment></comment>
  LowVoltageBatteryVoltage[V]___UNIQUE_1 : Outport  Description=|  Port=2  PortDimensions=[1]  VectorParamsAs1DForOutWhenUnconnected=off
      | <name>LowVoltageBattery.LowVoltageBatteryVoltage[V]</name>
      | <comment></comment>
  StarterVoltage[V]___UNIQUE_1 : Outport  Description=|  Port=3  PortDimensions=[1]  VectorParamsAs1DForOutWhenUnconnected=off
      | <name>StarterVoltage[V]</name>
      | <comment></comment>
  wires:
  __TDD__StarterVoltage[V]/1 -> StarterVoltage[V]___UNIQUE_1/1  "StarterVoltage[V]"
  __TDD__LowVoltageBatteryVoltage[V]/1 -> LowVoltageBatteryVoltage[V]___UNIQUE_1/1  "LowVoltageBatteryVoltage[V]"
  __TDD__GeneratorVoltage[V]/1 -> GeneratorVoltage[V]___UNIQUE_1/1  "GeneratorVoltage[V]"
  TDBusSelector/3 -> __TDD__StarterVoltage[V]/1  "<StarterVoltage[V]>"
  TDBusSelector/2 -> __TDD__LowVoltageBatteryVoltage[V]/1  "<LowVoltageBatteryVoltage[V]>"
  TDBusSelector/1 -> __TDD__GeneratorVoltage[V]/1  "<GeneratorVoltage[V]>"
  fromPowernet/1 -> TDBusSelector/1

== system SingleTrackCANoe/SimulationModel/Vehicle/Auxiliaries/SimpleEnergyManagement ==
  StarterSwitch [0;1] : Inport
  Generator off : Constant  Value=0
  GeneratorReferenceVoltage : LookupTableModules/ConstantVoltage  DATA_NODE=MDL.Vehicle.Auxiliaries.GeneratorReferenceVoltage  ConstVoltage=MDL.Vehicle.Auxiliaries.GeneratorReferenceVoltage.Voltage
  Switch : Switch  Threshold=0.5
  RefVoltage [V] : Outport  VectorParamsAs1DForOutWhenUnconnected=off
  wires:
  GeneratorReferenceVoltage/1 -> Switch/3
  Switch/1 -> RefVoltage [V]/1
  StarterSwitch [0;1]/1 -> Switch/2
  Generator off/1 -> Switch/1

== system SingleTrackCANoe/SimulationModel/Vehicle/Auxiliaries/Starter ==
  StarterVoltage [V] : Inport
  EngSpd [rad/s] : Inport  Port=2
  StarterSwitch [0;1] : Inport  Port=3
  Temp [K] : Inport  Port=4
  PermanentMagnetDCMotor : AuxiliariesModules/PermanentMagnetDCMotor  DATA_NODE=MDL.Vehicle.Auxiliaries.PermanentMagnetDCMotor  flux=MDL.Vehicle.Auxiliaries.PermanentMagnetDCMotor.FieldFlux  armature_inductance=MDL.Vehicle.Auxiliaries.PermanentMagnetDCMotor.ArmatureInduct  armature_resistance=MDL.Vehicle.Auxiliaries.PermanentMagnetDCMotor.ArmatureResistCurve  motor_const=MDL.Vehicle.Auxiliaries.PermanentMagnetDCMotor.MotorConst  inrt=MDL.Vehicle.Auxiliaries.PermanentMagnetDCMotor.Inrt  heat_cap=MDL.Vehicle.Auxiliaries.PermanentMagnetDCMotor.HeatCap
  StarterControl : AuxiliariesModules/StarterControl  DATA_NODE=MDL.Vehicle.Auxiliaries.StarterControl  speedratio=MDL.Vehicle.Auxiliaries.StarterControl.StarterEngSpdRatio
  Terminator : Terminator
  Terminator1 : Terminator
  Terminator2 : Terminator
  StarterCurr [A] : Outport  VectorParamsAs1DForOutWhenUnconnected=off
  StarterTrq [Nm] : Outport  Port=2  VectorParamsAs1DForOutWhenUnconnected=off
  StarterInrt [kgm**2] : Outport  Port=3  VectorParamsAs1DForOutWhenUnconnected=off
  wires:
  PermanentMagnetDCMotor/4 -> StarterControl/6
  StarterControl/1 -> StarterCurr [A]/1
  StarterControl/2 -> StarterTrq [Nm]/1
  StarterControl/3 -> StarterInrt [kgm**2]/1
  StarterControl/4 -> PermanentMagnetDCMotor/1
  StarterControl/5 -> PermanentMagnetDCMotor/3
  PermanentMagnetDCMotor/1 -> StarterControl/4
  StarterVoltage [V]/1 -> StarterControl/1
  EngSpd [rad/s]/1 -> StarterControl/3
  StarterSwitch [0;1]/1 -> StarterControl/2
  PermanentMagnetDCMotor/3 -> StarterControl/5
  Temp [K]/1 -> PermanentMagnetDCMotor/2
  PermanentMagnetDCMotor/2 -> Terminator/1
  PermanentMagnetDCMotor/5 -> Terminator1/1
  PermanentMagnetDCMotor/6 -> Terminator2/1

== system SingleTrackCANoe/SimulationModel/Vehicle/BrakeSystem/BrakeSystemControlUnit ==
  fromBrakeSystemPhysics : Inport
  fromCTRL : Inport  Port=2
  fromWheelSystem : Inport  Port=3
  fromChassis : Inport  Port=4
  BrakeSystemControlUnitOutput : Subsystem  Tag=TESIS DYNAware Interface Block  mask{NeedsUpdate=off, SignalInfo=|}
      mask SignalInfo=|
      | {
      |   "Version": "4.6",
      |   "MuxedOutputBusName": "BrakeSystemControlUnit",
      |   "MuxedInputBusName": "",
      |   "MuxedInputSelected": false,
      |   "MuxedOutputSelected": true,
      |   "SignalData": [
      |     {
      |       "initialValue": "0.0",
      |       "name": "",
      |       "comment": "Front left wheel brake pressure",
      |       "minString": "",
      |       "maxString": "",
      |       "width": 1,
      |       "dataType": 0,
      |       "signalType": 0,
      |       "createSignal": true,
      |       "outputName": "FrontLeftWheelBrakePress[Pa]",
      |       "generateSignalAccessBlock": false,
      |       "accessId": "$(parentId).$(blockName).$(outputName)"
      |     },
      |     {
      |       "initialValue": "0.0",
      |       "name": "",
      |       "comment": "Front right wheel brake pressure",
      |       "minString": "",
      |       "maxString": "",
      |       "width": 1,
      |       "dataType": 0,
      |       "signalType": 0,
      |       "createSignal": true,
      |       "outputName": "FrontRightWheelBrakePress[Pa]",
      |       "generateSignalAccessBlock": false,
      |       "accessId": "$(parentId).$(blockName).$(outputName)"
      |     },
      |     {
      |       "initialValue": "0.0",
      |       "name": "",
      |       "comment": "Rear left wheel brake pressure",
      |       "minString": "",
      |       "maxString": "",
      |       "width": 1,
      |       "dataType": 0,
      |       "signalType": 0,
      |       "createSignal": true,
      |       "outputName": "RearLeftWheelBrakePress[Pa]",
      |       "generateSignalAccessBlock": false,
      |       "accessId": "$(parentId).$(blockName).$(outputName)"
      |     },
      |     {
      |       "initialValue": "0.0",
      |       "name": "",
      |       "comment": "Rear right wheel brake pressure",
      |       "minString": "",
      |       "maxString": "",
      |       "width": 1,
      |       "dataType": 0,
      |       "signalType": 0,
      |       "createSignal": true,
      |       "outputName": "RearRightWheelBrakePress[Pa]",
      |       "generateSignalAccessBlock": false,
      |       "accessId": "$(parentId).$(blockName).$(outputName)"
      |     },
      |     {
      |       "initialValue": "0.0",
      |       "name": "",
      |       "comment": "",
      |       "minString": "",
      |       "maxString": "",
      |       "width": 1,
      |       "dataType": 0,
      |       "signalType": 0,
      |       "createSignal": true,
      |       "outputName": "Rear2LeftWheelBrakePress[Pa]",
      |       "generateSignalAccessBlock": false,
      |       "accessId": "$(parentId).$(blockName).$(outputName)"
      |     },
      |     {
      |       "initialValue": "0.0",
      |       "name": "",
      |       "comment": "",
      |       "minString": "",
      |       "maxString": "",
      |       "width": 1,
      |       "dataType": 0,
      |       "signalType": 0,
      |       "createSignal": true,
      |       "outputName": "Rear2RightWheelBrakePress[Pa]",
      |       "generateSignalAccessBlock": false,
      |       "accessId": "$(parentId).$(blockName).$(outputName)"
      |     },
      |     {
      |       "initialValue": "0.0",
      |       "name": "",
      |       "comment": "",
      |       "minString": "",
      |       "maxString": "",
      |       "width": 1,
      |       "dataType": 0,
      |       "signalType": 0,
      |       "createSignal": true,
      |       "outputName": "Rear3LeftWheelBrakePress[Pa]",
      |       "generateSignalAccessBlock": false,
      |       "accessId": "$(parentId).$(blockName).$(outputName)"
      |     },
      |     {
      |       "initialValue": "0.0",
      |       "name": "",
      |       "comment": "",
      |       "minString": "",
      |       "maxString": "",
      |       "width": 1,
      |       "dataType": 0,
      |       "signalType": 0,
      |       "createSignal": true,
      |       "outputName": "Rear3RightWheelBrakePress[Pa]",
      |       "generateSignalAccessBlock": false,
      |       "accessId": "$(parentId).$(blockName).$(outputName)"
      |     },
      |     {
      |       "initialValue": "0.0",
      |       "name": "",
      |       "comment": "",
      |       "minString": "",
      |       "maxString": "",
      |       "width": 1,
      |       "dataType": 0,
      |       "signalType": 0,
      |       "createSignal": true,
      |       "outputName": "WheelBrakePressActive[0;1]",
      |       "generateSignalAccessBlock": false,
      |       "accessId": "$(parentId).$(blockName).$(outputName)"
      |     },
      |     {
      |       "initialValue": "0.0",
      |       "name": "",
      |       "comment": "",
      |       "minString": "",
      |       "maxString": "",
      |       "width": -1,
      |       "dataType": 0,
      |       "signalType": 1,
      |       "createSignal": true,
      |       "outputName": "ControlUnit",
      |       "generateSignalAccessBlock": false,
      |       "accessId": "$(parentId).$(blockName).$(outputName)"
      |     }
      |   ]
      | }
      mask prompts: NeedsUpdate "Specify, if subsystem content needs to be updated"; SignalInfo "Signal Info (json)"
      mask help: DYNA4 Interface Block Version 4.6
      mask init:
      | blockName = get_param(gcbh, 'Name');
      | parentId = DYNA4.ModelHandling.AccessID.getFromHierarchy(gcbh);
      | TD.InterfaceBlock.ModelCallbacks.GenerateContent(gcb);
      settings: DeleteFcn=TD.InterfaceBlock.ModelCallbacks.CloseGUI( gcbh );  NameChangeFcn=TD.InterfaceBlock.ModelCallbacks.BlockRenamedHandler(gcbh);  OpenFcn=TD.InterfaceBlock.ModelCallbacks.OpenGUI( gcbh );  CloseFcn=TD.InterfaceBlock.ModelCallbacks.CloseGUI( gcbh );
      settings: AttributesFormatString=|
      | FrontLeftWheelBrakePress[Pa] = 0.0
      | FrontRightWheelBrakePress[Pa] = 0.0
      | RearLeftWheelBrakePress[Pa] = 0.0
      | RearRightWheelBrakePress[Pa] = 0.0
      | ...
      mask Display:
      | image('InterfaceBlock.png','center');
      | port_label('output',1, 'BrakeSystemControlUnit');
  DynaComponentInfo : Subsystem  Tag=DynaComponentInfo
      mask init:
      | data= get_param(gcb, 'UserData');
      settings: OpenFcn=DYNA4.ModelHandling.Component.ShowEditComponentInformationDialog(gcb);
      mask Display: disp(['Type = ', data.type, '\nGroup = ', data.group, '\nName = ', data.name ])
  Terminator{1..4} (4 alike) : Terminator
  BrakeSystemControlUnit : Outport  VectorParamsAs1DForOutWhenUnconnected=off
  wires:
  BrakeSystemControlUnitOutput/1(BrakeSystemControlUnit___UNIQUE_1) -> BrakeSystemControlUnit/1
  fromBrakeSystemPhysics/1 -> Terminator4/1
  fromCTRL/1 -> Terminator1/1
  fromChassis/1 -> Terminator3/1
  fromWheelSystem/1 -> Terminator2/1

== system SingleTrackCANoe/SimulationModel/Vehicle/BrakeSystem/BrakeSystemOutputs ==
  BrakeSystemPhysics___UNIQUE_1 : Inport  Description=|
      | <name>BrakeSystemPhysics</name>
      | <comment></comment>
  BrakeSystemControlUnitInfo___UNIQUE_1 : Inport  Description=|  Port=2
      | <name>BrakeSystemControlUnitInfo</name>
      | <comment></comment>
  __TDO__BrakeSystem : BusCreator  Inputs=2
  BrakeSystem___UNIQUE_1 : Outport  Description=|  VectorParamsAs1DForOutWhenUnconnected=off
      | <name>BrakeSystemPhysics</name>
      | <comment></comment>
  wires:
  __TDO__BrakeSystem/1 -> BrakeSystem___UNIQUE_1/1  "BrakeSystem"
  BrakeSystemControlUnitInfo___UNIQUE_1/1 -> __TDO__BrakeSystem/2  "BrakeSystemControlUnitInfo"
  BrakeSystemPhysics___UNIQUE_1/1 -> __TDO__BrakeSystem/1  "BrakeSystemPhysics"

== system SingleTrackCANoe/SimulationModel/Vehicle/BrakeSystem/BrakeSystemPhysics ==
  fromBrakeControlCoordinator : Inport
  fromCTRL : Inport  Port=2
  fromBrakeSystemControlUnit : Inport  Port=3
  BrakeSystemPhysicsOutput : Subsystem  Tag=TESIS DYNAware Interface Block  mask{NeedsUpdate=off, SignalInfo=|}
      mask SignalInfo=|
      | {
      |   "Version": "4.6",
      |   "MuxedOutputBusName": "BrakeSystemPhysics",
      |   "MuxedInputBusName": "input",
      |   "MuxedInputSelected": false,
      |   "MuxedOutputSelected": true,
      |   "SignalData": [
      |     {
      |       "initialValue": "0.0",
      |       "name": "WheelBrakePressActive[0;1]",
      |       "comment": "",
      |       "minString": "",
      |       "maxString": "",
      |       "width": 1,
      |       "dataType": 0,
      |       "signalType": 0,
      |       "createSignal": false,
      |       "outputName": "WheelBrakePressActive[0;1]",
      |       "generateSignalAccessBlock": false,
      |       "accessId": "$(parentId).$(blockName).$(outputName)"
      |     },
      |     {
      |       "initialValue": "0.0",
      |       "name": "MaxMainBrakePress[Pa]",
      |       "comment": "",
      |       "minString": "",
      |       "maxString": "",
      |       "width": 1,
      |       "dataType": 0,
      |       "signalType": 0,
      |       "createSignal": false,
      |       "outputName": "MaxMainBrakePress[Pa]",
      |       "generateSignalAccessBlock": false,
      |       "accessId": "$(parentId).$(blockName).$(outputName)"
      |     },
      |     {
      |       "initialValue": "0.0",
      |       "name": "MainBrakePress[Pa]",
      |       "comment": "",
      |       "minString": "",
      |       "maxString": "",
      |       "width": 1,
      |       "dataType": 0,
      |       "signalType": 0,
      |       "createSignal": false,
      |       "outputName": "MainBrakePress[Pa]",
      |       "generateSignalAccessBlock": false,
      |       "accessId": "$(parentId).$(blockName).$(outputName)"
      |     },
      |     {
      |       "initialValue": "",
      |       "name": "FrontLeftWheelBrakePress[Pa]",
      |       "comment": "",
      |       "minString": "",
      |       "maxString": "",
      |       "width": 1,
      |       "dataType": 0,
      |       "signalType": 0,
      |       "createSignal": false,
      |       "outputName": "FrontLeftWheelBrakePress[Pa]",
      |       "generateSignalAccessBlock": false,
      |       "accessId": "$(parentId).$(blockName).$(outputName)"
      |     },
      |     {
      |       "initialValue": "",
      |       "name": "FrontRightWheelBrakePress[Pa]",
      |       "comment": "",
      |       "minString": "",
      |       "maxString": "",
      |       "width": 1,
      |       "dataType": 0,
      |       "signalType": 0,
      |       "createSignal": false,
      |       "outputName": "FrontRightWheelBrakePress[Pa]",
      |       "generateSignalAccessBlock": false,
      |       "accessId": "$(parentId).$(blockName).$(outputName)"
      |     },
      |     {
      |       "initialValue": "",
      |       "name": "RearLeftWheelBrakePress[Pa]",
      |       "comment": "",
      |       "minString": "",
      |       "maxString": "",
      |       "width": 1,
      |       "dataType": 0,
      |       "signalType": 0,
      |       "createSignal": false,
      |       "outputName": "RearLeftWheelBrakePress[Pa]",
      |       "generateSignalAccessBlock": false,
      |       "accessId": "$(parentId).$(blockName).$(outputName)"
      |     },
      |     {
      |       "initialValue": "",
      |       "name": "RearRightWheelBrakePress[Pa]",
      |       "comment": "",
      |       "minString": "",
      |       "maxString": "",
      |       "width": 1,
      |       "dataType": 0,
      |       "signalType": 0,
      |       "createSignal": false,
      |       "outputName": "RearRightWheelBrakePress[Pa]",
      |       "generateSignalAccessBlock": false,
      |       "accessId": "$(parentId).$(blockName).$(outputName)"
      |     },
      |     {
      |       "initialValue": "",
      |       "name": "Rear2LeftWheelBrakePress[Pa]",
      |       "comment": "",
      |       "minString": "",
      |       "maxString": "",
      |       "width": 1,
      |       "dataType": 0,
      |       "signalType": 0,
      |       "createSignal": false,
      |       "outputName": "Rear2LeftWheelBrakePress[Pa]",
      |       "generateSignalAccessBlock": false,
      |       "accessId": "$(parentId).$(blockName).$(outputName)"
      |     },
      |     {
      |       "initialValue": "",
      |       "name": "Rear2RightWheelBrakePress[Pa]",
      |       "comment": "",
      |       "minString": "",
      |       "maxString": "",
      |       "width": 1,
      |       "dataType": 0,
      |       "signalType": 0,
      |       "createSignal": false,
      |       "outputName": "Rear2RightWheelBrakePress[Pa]",
      |       "generateSignalAccessBlock": false,
      |       "accessId": "$(parentId).$(blockName).$(outputName)"
      |     },
      |     {
      |       "initialValue": "",
      |       "name": "Rear3LeftWheelBrakePress[Pa]",
      |       "comment": "",
      |       "minString": "",
      |       "maxString": "",
      |       "width": 1,
      |       "dataType": 0,
      |       "signalType": 0,
      |       "createSignal": false,
      |       "outputName": "Rear3LeftWheelBrakePress[Pa]",
      |       "generateSignalAccessBlock": false,
      |       "accessId": "$(parentId).$(blockName).$(outputName)"
      |     },
      |     {
      |       "initialValue": "",
      |       "name": "Rear3RightWheelBrakePress[Pa]",
      |       "comment": "",
      |       "minString": "",
      |       "maxString": "",
      |       "width": 1,
      |       "dataType": 0,
      |       "signalType": 0,
      |       "createSignal": false,
      |       "outputName": "Rear3RightWheelBrakePress[Pa]",
      |       "generateSignalAccessBlock": false,
      |       "accessId": "$(parentId).$(blockName).$(outputName)"
      |     }
      |   ]
      | }
      mask prompts: NeedsUpdate "Specify, if subsystem content needs to be updated"; SignalInfo "Signal Info (json)"
      mask help: DYNA4 Interface Block Version 4.6
      mask init:
      | blockName = get_param(gcbh, 'Name');
      | parentId = DYNA4.ModelHandling.AccessID.getFromHierarchy(gcbh);
      | TD.InterfaceBlock.ModelCallbacks.GenerateContent(gcb);
      settings: DeleteFcn=TD.InterfaceBlock.ModelCallbacks.CloseGUI( gcbh );  NameChangeFcn=TD.InterfaceBlock.ModelCallbacks.BlockRenamedHandler(gcbh);  OpenFcn=TD.InterfaceBlock.ModelCallbacks.OpenGUI( gcbh );  CloseFcn=TD.InterfaceBlock.ModelCallbacks.CloseGUI( gcbh );
      mask Display:
      | image('InterfaceBlock.png','center');
      | port_label('input',1, 'WheelBrakePressActive[0;1]');
      | port_label('input',2, 'MaxMainBrakePress[Pa]');
      | port_label('input',3, 'MainBrakePress[Pa]');
      | port_label('input',4, 'FrontLeftWheelBrakePress[Pa]');
      | port_label('input',5, 'FrontRightWheelBrakePress[Pa]');
      | port_label('input',6, 'RearLeftWheelBrakePress[Pa]');
      | port_label('input',7, 'RearRightWheelBrakePress[Pa]');
      | port_label('input',8, 'Rear2LeftWheelBrakePress[Pa]');
      | port_label('input',9, 'Rear2RightWheelBrakePress[Pa]');
      | port_label('input',10, 'Rear3LeftWheelBrakePress[Pa]');
      | port_label('input',11, 'Rear3RightWheelBrakePress[Pa]');
      | port_label('output',1, 'BrakeSystemPhysics');
  Compare To Constant : simulink/Logic and Bit Operations/Compare To Constant  relop=~=  const=double(DYNA4.Vehicle.BrakeSystem.BrakeSwitch.WHEEL_BRAKE_PRESSURES)  OutDataTypeStr=boolean
  Data Type Conversion : DataTypeConversion  OutDataTypeStr=double
  Demux : Demux  Outputs=8
  DynaComponentInfo : Subsystem  Tag=DynaComponentInfo
      mask init:
      | data= get_param(gcb, 'UserData');
      settings: OpenFcn=DYNA4.ModelHandling.Component.ShowEditComponentInformationDialog(gcb);
      mask Display: disp(['Type = ', data.type, '\nGroup = ', data.group, '\nName = ', data.name ])
  InputFromBrakeControlCoordinator : Subsystem  Tag=TESIS DYNAware Interface Block  mask{NeedsUpdate=off, SignalInfo=|}
      mask SignalInfo=|
      | {
      |   "Version": "4.6",
      |   "MuxedOutputBusName": "output",
      |   "MuxedInputBusName": "fromBrakeControlCoordinator",
      |   "MuxedInputSelected": true,
      |   "MuxedOutputSelected": false,
      |   "SignalData": [
      |     {
      |       "initialValue": "",
      |       "name": "BrakeSwitch[1;3]",
      |       "comment": "",
      |       "minString": "",
      |       "maxString": "",
      |       "width": -1,
      |       "dataType": 0,
      |       "signalType": 0,
      |       "createSignal": false,
      |       "outputName": "BrakeSwitch[1;3]",
      |       "generateSignalAccessBlock": false,
      |       "accessId": "$(parentId).$(blockName).$(outputName)"
      |     },
      |     {
      |       "initialValue": "",
      |       "name": "MainBrakePress[Pa]",
      |       "comment": "",
      |       "minString": "",
      |       "maxString": "",
      |       "width": -1,
      |       "dataType": 0,
      |       "signalType": 0,
      |       "createSignal": false,
      |       "outputName": "MainBrakePress[Pa]",
      |       "generateSignalAccessBlock": false,
      |       "accessId": "$(parentId).$(blockName).$(outputName)"
      |     }
      |   ]
      | }
      mask prompts: NeedsUpdate "Specify, if subsystem content needs to be updated"; SignalInfo "Signal Info (json)"
      mask help: DYNA4 Interface Block Version 4.6
      mask init:
      | blockName = get_param(gcbh, 'Name');
      | parentId = DYNA4.ModelHandling.AccessID.getFromHierarchy(gcbh);
      | TD.InterfaceBlock.ModelCallbacks.GenerateContent(gcb);
      settings: DeleteFcn=TD.InterfaceBlock.ModelCallbacks.CloseGUI( gcbh );  NameChangeFcn=TD.InterfaceBlock.ModelCallbacks.BlockRenamedHandler(gcbh);  OpenFcn=TD.InterfaceBlock.ModelCallbacks.OpenGUI( gcbh );  CloseFcn=TD.InterfaceBlock.ModelCallbacks.CloseGUI( gcbh );
      mask Display:
      | image('InterfaceBlock.png','center');
      | port_label('input',1, 'fromBrakeControlCoordinator');
      | port_label('output',1, 'BrakeSwitch[1;3]');
      | port_label('output',2, 'MainBrakePress[Pa]');
  InputFromCTRL : Subsystem  Tag=TESIS DYNAware Interface Block  mask{NeedsUpdate=off, SignalInfo=|}
      mask SignalInfo=|
      | {
      |   "Version": "4.6",
      |   "MuxedOutputBusName": "output",
      |   "MuxedInputBusName": "fromCTRL",
      |   "MuxedInputSelected": true,
      |   "MuxedOutputSelected": false,
      |   "SignalData": {
      |     "initialValue": "0.0",
      |     "name": "CTRL.LongitudinalControl.BrakePedalPos[0_1]",
      |     "comment": "",
      |     "minString": "",
      |     "maxString": "",
      |     "width": 1,
      |     "dataType": 0,
      |     "signalType": 0,
      |     "createSignal": false,
      |     "outputName": "BrakePedalPos[0_1]",
      |     "generateSignalAccessBlock": false,
      |     "accessId": "$(parentId).$(blockName).$(outputName)"
      |   }
      | }
      mask prompts: NeedsUpdate "Specify, if subsystem content needs to be updated"; SignalInfo "Signal Info (json)"
      mask help: DYNA4 Interface Block Version 4.6
      mask init:
      | blockName = get_param(gcbh, 'Name');
      | parentId = DYNA4.ModelHandling.AccessID.getFromHierarchy(gcbh);
      | TD.InterfaceBlock.ModelCallbacks.GenerateContent(gcb);
      settings: DeleteFcn=TD.InterfaceBlock.ModelCallbacks.CloseGUI( gcbh );  NameChangeFcn=TD.InterfaceBlock.ModelCallbacks.BlockRenamedHandler(gcbh);  OpenFcn=TD.InterfaceBlock.ModelCallbacks.OpenGUI( gcbh );  CloseFcn=TD.InterfaceBlock.ModelCallbacks.CloseGUI( gcbh );
      mask Display:
      | image('InterfaceBlock.png','center');
      | port_label('input',1, 'fromCTRL');
      | port_label('output',1, 'BrakePedalPos[0_1]');
  TabledBrakeHydraulics : BrakeSystemModules/TabledBrakeHydraulics  Tag=vedynaBrkHydMask  local_comp_inst=1  system_comp_inst=1  DATA_NODE=MDL.Vehicle.BrakeSystem.BrakeSystemPhysics.TabledBrakeHydraulics  sample_time=-1
  Terminator : Terminator
  BrakeSystemPhysics : Outport  VectorParamsAs1DForOutWhenUnconnected=off
  wires:
  Demux/1 -> BrakeSystemPhysicsOutput/4(FrontLeftWheelBrakePress[Pa]___UNIQUE_1)
  Demux/2 -> BrakeSystemPhysicsOutput/5(FrontRightWheelBrakePress[Pa]___UNIQUE_1)
  Demux/3 -> BrakeSystemPhysicsOutput/6(RearLeftWheelBrakePress[Pa]___UNIQUE_1)
  Demux/4 -> BrakeSystemPhysicsOutput/7(RearRightWheelBrakePress[Pa]___UNIQUE_1)
  Demux/5 -> BrakeSystemPhysicsOutput/8(Rear2LeftWheelBrakePress[Pa]___UNIQUE_1)
  Demux/6 -> BrakeSystemPhysicsOutput/9(Rear2RightWheelBrakePress[Pa]___UNIQUE_1)
  Demux/7 -> BrakeSystemPhysicsOutput/10(Rear3LeftWheelBrakePress[Pa]___UNIQUE_1)
  Demux/8 -> BrakeSystemPhysicsOutput/11(Rear3RightWheelBrakePress[Pa]___UNIQUE_1)
  InputFromCTRL/1(BrakePedalPos[0_1]___UNIQUE_1) -> TabledBrakeHydraulics/2
  fromCTRL/1 -> InputFromCTRL/1(fromCTRL)
  TabledBrakeHydraulics/3 -> Demux/1
  TabledBrakeHydraulics/2 -> BrakeSystemPhysicsOutput/3(MainBrakePress[Pa]___UNIQUE_1)
  TabledBrakeHydraulics/1 -> BrakeSystemPhysicsOutput/2(MaxMainBrakePress[Pa]___UNIQUE_1)
  BrakeSystemPhysicsOutput/1(BrakeSystemPhysics___UNIQUE_1) -> BrakeSystemPhysics/1
  fromBrakeControlCoordinator/1 -> InputFromBrakeControlCoordinator/1(fromBrakeControlCoordinator)
  InputFromBrakeControlCoordinator/1(BrakeSwitch[1;3]___UNIQUE_1) -> TabledBrakeHydraulics/1, Compare To Constant/1
  InputFromBrakeControlCoordinator/2(MainBrakePress[Pa]___UNIQUE_1) -> TabledBrakeHydraulics/3
  fromBrakeSystemControlUnit/1 -> Terminator/1
  Compare To Constant/1 -> Data Type Conversion/1
  Data Type Conversion/1 -> BrakeSystemPhysicsOutput/1(WheelBrakePressActive[0;1]___UNIQUE_1)
